simulink model "Lab05"  (R2024b)
settings: Solver=ode8  StartTime=0.0  StopTime=tf  FixedStep=0.025  RelTol=1e-3
values from neighbouring files (symbols this model uses):
  I = diag(Iv)    [initLab5.m]
  invI = inv(I)    [initLab5.m]
  w0 = [0.45; 0.52; 0.55]    [initLab5.m]
undefined symbols (not defined in the file or in its folder): IC
libraries: matrix_library x1
(part 4 of 4)

== system Lab05/Ordinato/A313 ==
  In1 : Inport
  Cos : Trigonometry  Operator=cos
  Cos1 : Trigonometry  Operator=cos
  Cos2 : Trigonometry  Operator=cos
  Demux : Demux  Outputs=3
  Gain : Gain  Gain=-1
  Matrix Concatenate : Concatenate  NumInputs=3  Mode=Multidimensional array
  Matrix Concatenate1 : Concatenate  NumInputs=3  Mode=Multidimensional array
  Matrix Concatenate3 : Concatenate  NumInputs=3  Mode=Multidimensional array  ConcatenateDimension=2
  Matrix Concatenate4 : Concatenate  NumInputs=3  Mode=Multidimensional array
  Product{1,3,5..6,8,10..12} (8 alike) : Product
  Product{2,4,7,9} (4 alike) : Product  Inputs=3
  Sin : Trigonometry
  Sin1 : Trigonometry
  Sin2 : Trigonometry
  Subtract : Sum  Inputs=+-
  Subtract1 : Sum  Inputs=--
  Subtract2 : Sum
  Subtract3 : Sum  Inputs=-+
  Out1 : Outport
  wires:
  In1/1 -> Demux/1
  [cosTheta] -> Product2/3
  Product7/1 -> Subtract2/2
  [sinTheta] -> Product11/2
  [sinPhi] -> Product8/2
  Sin/1 -> [sinPhi]
  [cosTheta] -> Product4/3
  [sinPhi] -> Product2/2
  [sinTheta] -> Product10/2
  Product5/1 -> Matrix Concatenate/3
  [cosPsi] -> Product6/1
  Demux/3 -> Sin2/1, Cos2/1
  Product9/1 -> Subtract3/2
  [cosTheta] -> Matrix Concatenate1/3
  Matrix Concatenate1/1 -> Matrix Concatenate3/3
  [sinPsi] -> Product11/1
  Product2/1 -> Subtract/2
  [sinPhi] -> Product4/2
  Subtract2/1 -> Matrix Concatenate4/1
  Matrix Concatenate4/1 -> Matrix Concatenate3/2
  [cosPsi] -> Product12/1
  Cos2/1 -> [cosPsi]
  Product10/1 -> Gain/1
  [sinPsi] -> Product2/1
  [sinPsi] -> Product8/1
  Sin2/1 -> [sinPsi]
  [cosTheta] -> Product7/3
  Subtract/1 -> Matrix Concatenate/1
  [cosPhi] -> Product10/1
  Subtract1/1 -> Matrix Concatenate/2
  Subtract3/1 -> Matrix Concatenate4/2
  Demux/2 -> Sin1/1, Cos1/1
  [cosTheta] -> Product9/3
  Product8/1 -> Subtract3/1
  [cosPhi] -> Product9/2
  [cosPsi] -> Product9/1
  Gain/1 -> Matrix Concatenate4/3
  [cosPsi] -> Product4/1
  Product11/1 -> Matrix Concatenate1/1
  Product1/1 -> Subtract/1
  [cosPhi] -> Product1/2
  [sinTheta] -> Product12/2
  [cosPhi] -> Product7/2
  [sinPhi] -> Product6/2
  Product6/1 -> Subtract2/1
  Demux/1 -> Sin/1, Cos/1
  [cosPsi] -> Product1/1
  [sinPsi] -> Product7/1
  Cos1/1 -> [cosTheta]
  Sin1/1 -> [sinTheta]
  [sinTheta] -> Product5/2
  [sinPsi] -> Product3/1
  Product12/1 -> Matrix Concatenate1/2
  [sinPhi] -> Product5/1
  Product3/1 -> Subtract1/1
  Product4/1 -> Subtract1/2
  [cosPhi] -> Product3/2
  Matrix Concatenate/1 -> Matrix Concatenate3/1
  Cos/1 -> [cosPhi]
  Matrix Concatenate3/1 -> Out1/1

== system Lab05/Quaternions/Omega ==
  In1 : Inport
  Constant{,1..3} (4 alike) : Constant  Value=0
  Demux : Demux  Outputs=3
  Gain{,1..5} (6 alike) : Gain  Gain=-1
  Matrix Concatenate{,1..3} (4 alike) : Concatenate  NumInputs=4  Mode=Multidimensional array
  Matrix Concatenate4 : Concatenate  NumInputs=4  Mode=Multidimensional array  ConcatenateDimension=2
  Out1 : Outport
  wires:
  In1/1 -> Demux/1
  Demux/1 -> [wx]
  Demux/2 -> [wy]
  Demux/3 -> [wz]
  Matrix Concatenate1/1 -> Matrix Concatenate4/1
  Matrix Concatenate2/1 -> Matrix Concatenate4/2
  Matrix Concatenate/1 -> Matrix Concatenate4/4
  Matrix Concatenate3/1 -> Matrix Concatenate4/3
  Constant/1 -> Matrix Concatenate1/1
  Constant1/1 -> Matrix Concatenate2/2
  Constant2/1 -> Matrix Concatenate3/3
  Constant3/1 -> Matrix Concatenate/4
  Gain/1 -> Matrix Concatenate3/1
  Gain1/1 -> Matrix Concatenate3/4
  Gain2/1 -> Matrix Concatenate2/4
  Gain3/1 -> Matrix Concatenate2/3
  Gain4/1 -> Matrix Concatenate1/4
  Gain5/1 -> Matrix Concatenate1/2
  [wz] -> Gain5/1
  [wz] -> Matrix Concatenate2/1
  [wz] -> Gain1/1
  [wz] -> Matrix Concatenate/3
  [wy] -> Matrix Concatenate1/3
  [wz] -> Gain2/1
  [wz] -> Gain/1
  [wz] -> Matrix Concatenate/2
  Matrix Concatenate4/1 -> Out1/1
  [wx] -> Gain4/1
  [wx] -> Gain3/1
  [wx] -> Matrix Concatenate3/2
  [wx] -> Matrix Concatenate/1
